simulink model "RocketThrottlingControllersSimulink"  (R2025b)
settings: Solver=ode4  StartTime=0.0  StopTime=6  FixedStep=1e-4  MaxStep=1e-3  RelTol=1e-6
libraries: slpidlib x3, mpclib x2
settings Model: ExtModeTrigDuration=2  Creator=marietakysela  LastModifiedBy=marietakysela
settings SolverCC: AutoInsertRateTranBlk=on
settings OptimizationCC: EnhancedBackFolding=on  PassReuseOutputArgsAs=Individual arguments  ZeroExternalMemoryAtStartup=off  ZeroInternalMemoryAtStartup=off  MaxStackSize=64  OptimizeBlockOrder=speed  DifferentSizesBufferReuse=on  EfficientTunableParamExpr=on
settings DebuggingCC: ParameterTunabilityLossMsg=error
settings HardwareCC: ProdBitPerPointer=32.0  ProdBitPerSizeT=32.0  ProdBitPerPtrDiffT=32.0  ProdLargestAtomicInteger=Long  ProdLargestAtomicFloat=Double  ProdWordSize=32.0  ProdHWDeviceType=ARM Compatible->ARM Cortex  UseEmbeddedCoderFeatures=off  UseSimulinkCoderFeatures=off
settings SFSimCC: MATLABDynamicMemAlloc=off
settings RTWCC: SystemTargetFile=ert.tlc  HardwareBoard=Arduino Uno R4 WiFi  TemplateMakefile=ert_default_tmf  Toolchain=Arduino ARM M4  Description=Embedded Coder
settings CodeAppCC: ForceParamTrailComments=on  IgnoreCustomStorageClasses=off  OperatorAnnotations=on  SimulinkDataObjDesc=on  SFDataObjDesc=on  InsertBlockDesc=on
settings ERTTargetCC: ExtModeTransport=3.0  ExtModeStaticAlloc=on  ExtModeAutomaticAllocSize=off  ExtModeStaticAllocSize=8192.0  ExtModeMexFile=ext_xcp  ExtModeIntrfLevel=Level2 - Open  InlinedParameterPlacement=Hierarchical  SupportContinuousTime=on  SupportNonInlinedSFcns=on  SupportVariableSizeSignals=on

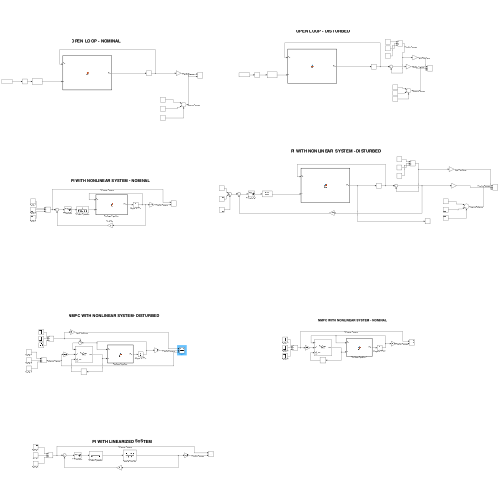
[thumbnail: Simulink's stored preview of the top-level diagram]
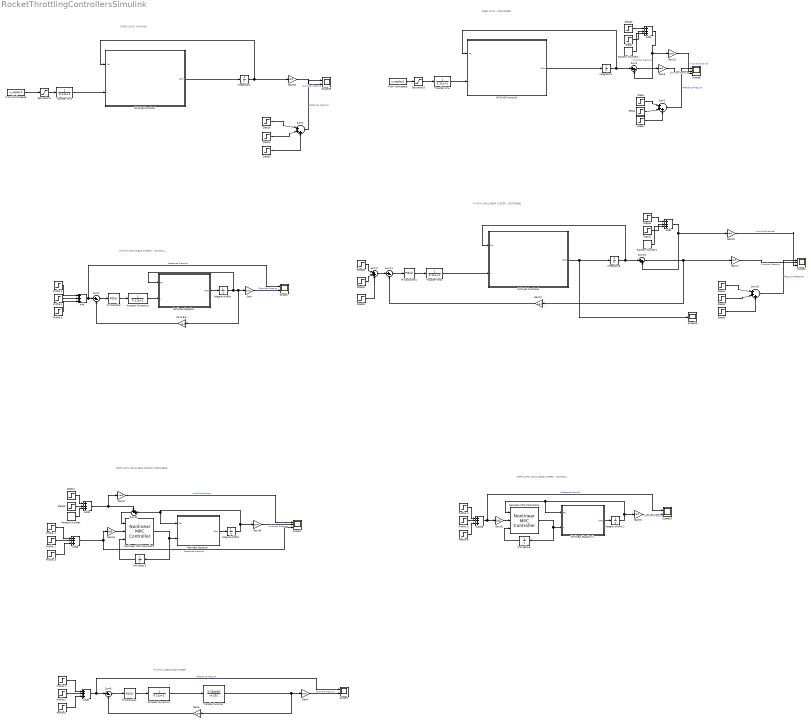
== system RocketThrottlingControllersSimulink ==
  note: PI WITH LINEARIZED SYSTEM
  note: PI WITH NONLINEAR SYSTEM - NOMINAL
  note: OPEN LOOP - DISTURBED
  note: PI WITH NONLINEAR SYSTEM - DISTURBED
  note: NMPC WITH NONLINEAR SYSTEM - NOMINAL
  note: NMPC WITH NONLINEAR SYSTEM- DISTURBED
  note: OPEN LOOP - NOMINAL
  .Integral of dPtc. : Integrator
  Actuator Dynamics : TransferFcn  Denominator=[0.11 1]
  Actuator Dynamics. : TransferFcn  Denominator=[0.11 1]
  Add{,1..2,6,8..9,16} (7 alike) : Sum  Inputs=+++
  From Workspace : FromWorkspace  VariableName=u_replay1
  From Workspace3 : FromWorkspace  VariableName=u_replay1
  Gain{,4..6,11..12,17..18,20..21,30,33} (12 alike) : Gain  Gain=1e-5
  Gain19 : Gain  Gain=1e5
  Gain31 : Gain  Gain=1e5
  Integral of dPtc : Integrator
  Integral of dPtc.2 : Integrator
  Integrator1 : Integrator
  Integrator2 : Integrator
  Integrator6 : Integrator
  MATLAB Function1 : MATLAB Function  TreatAsAtomicUnit=on
  MATLAB Function2 : MATLAB Function  TreatAsAtomicUnit=on
  MATLAB Function6 : MATLAB Function  TreatAsAtomicUnit=on
  "Nonlinear Equation " : MATLAB Function  TreatAsAtomicUnit=on
  Nonlinear Equation. : MATLAB Function  TreatAsAtomicUnit=on
  Nonlinear Equation.1 : MATLAB Function  TreatAsAtomicUnit=on
  Nonlinear MPC Controller3 : mpclib/Nonlinear MPC Controller  nlmpcobj=nlobj  UseObjectTs=on  UseMEX=off  md_enabled=off  mvtarget_enabled=off  param_enabled=off  cost_enabled=off  mvseq_enabled=off  stateseq_enabled=off  ovseq_enabled=off  slack_enabled=off  status_enabled=off  ov_min=off  ov_max=off  mv_min=off  mv_max=off  mvrate_min=off  mvrate_max=off  state_min=off  state_max=off  ov_weight=off  mv_weight=off  mvrate_weight=off  ecr_weight=off  nlp_initialize=off
  Nonlinear MPC Controller6 : mpclib/Nonlinear MPC Controller  nlmpcobj=nlobj  UseObjectTs=on  UseMEX=off  md_enabled=off  mvtarget_enabled=off  param_enabled=off  cost_enabled=off  mvseq_enabled=off  stateseq_enabled=off  ovseq_enabled=off  slack_enabled=off  status_enabled=off  ov_min=off  ov_max=off  mv_min=off  mv_max=off  mvrate_min=off  mvrate_max=off  state_min=off  state_max=off  ov_weight=off  mv_weight=off  mvrate_weight=off  ecr_weight=off  nlp_initialize=off
  PI Controller : slpidlib/PID Controller  Controller=PID  Form=Parallel  TimeDomain=Continuous-time  UseExternalTs=off  SampleTime=-1  IntegratorMethod=Forward Euler  FilterMethod=Forward Euler  ControllerParametersSource=internal  P=0.12  I=0.9  UseKiTs=off  D=0  UseExternalDerivativeSource=off  N=100  UseFilter=on  TunerSelectOption=Frequency Response Based  InitialConditionSource=internal  InitialConditionForIntegrator=0  InitialConditionForFilter=0  DifferentiatorICPrevScaledInput=0  ExternalReset=none  TrackingMode=off  Kt=1  LimitOutput=on  SatLimitsSource=internal  UpperSaturationLimit=0.5  LowerSaturationLimit=0  LinearizeAsGain=on  AntiWindupMode=back-calculation  Kb=8  LimitIntegrator=off  UpperIntegratorSaturationLimit=inf  LowerIntegratorSaturationLimit=-inf  POutMin=[]  POutMax=[]  IOutMin=[]  IOutMax=[]  DOutMin=[]  DOutMax=[]  NOutMin=[]  NOutMax=[]  SumOutMin=[]  SumOutMax=[]  SaturationOutMin=[]  SaturationOutMax=[]  PParamMin=[]  PParamMax=[]  IParamMin=[]  IParamMax=[]  DParamMin=[]  DParamMax=[]  NParamMin=[]  NParamMax=[]  KbParamMin=[]  KbParamMax=[]  KtParamMin=[]  KtParamMax=[]  KbOutMin=[]  KbOutMax=[]  KtOutMin=[]  KtOutMax=[]  IntegratorOutMin=[]  IntegratorOutMax=[]  FilterOutMin=[]  FilterOutMax=[]  SumI1OutMin=[]  SumI1OutMax=[]  SumI2OutMin=[]  SumI2OutMax=[]  SumI3OutMin=[]  SumI3OutMax=[]  SumI4OutMin=[]  SumI4OutMax=[]  SumDOutMin=[]  SumDOutMax=[]  DifferentiatorOutMin=[]  DifferentiatorOutMax=[]  FilterDiffOutCoefMin=[]  FilterDiffOutCoefMax=[]  ReciprocalOutMin=[]  ReciprocalOutMax=[]  SumDenOutMin=[]  SumDenOutMax=[]  SumNumOutMin=[]  SumNumOutMax=[]  DivideOutMin=[]  DivideOutMax=[]  UdiffTsProdOutMin=[]  UdiffTsProdOutMax=[]  NTsProdOutMin=[]  NTsProdOutMax=[]  UintegralTsProdOutMin=[]  UintegralTsProdOutMax=[]  UngainTsProdOutMin=[]  UngainTsProdOutMax=[]  ClampingZeroOutDataTypeStr=Inherit: Inherit via back propagation  ClampingZeroOutMin=[]  ClampingZeroOutMax=[]  FilterDenConstantOutDataTypeStr=Inherit: Inherit via back propagation  FilterDenConstantOutMin=[]  FilterDenConstantOutMax=[]  PCopyOutDataTypeStr=Inherit: Inherit via back propagation  PCopyOutMin=[]  PCopyOutMax=[]  NCopyOutDataTypeStr=Inherit: Inherit via back propagation  NCopyOutMin=[]  NCopyOutMax=[]  IntegratorContinuousStateAttributes=''  IntegratorStateMustResolveToSignalObject=off  IntegratorRTWStateStorageClass=Auto  FilterContinuousStateAttributes=''  FilterStateMustResolveToSignalObject=off  FilterRTWStateStorageClass=Auto  ParallelPVariant=InternalParameters  IdealPVariant=Disabled  IVariant=InternalParameters  DVariant=InternalParameters  IntegratorVariant=Continuous  SatVariant=Enabled  AWVariant=BackCalculation  PCopyVariant=Disabled  TRVariant=Disabled  FdbkBlocksVariant=Forward  IdealPFdbkVariant=Disabled  SatFdbkVariant=Disabled  DerivativeFilterVariant=ContFilter  NVariant=InternalParameters  NCopyVariant=Disabled  FilterICVariant=InternalICsFilter  IntegratorICVariant=InternalICs  ExternalResetVariant=Disabled  TRSumVariant=Passthrough  SumFdbkVariant=Disabled  SumVariant=Sum_PID  TsampFilterVariant=InternalTs  TsampNgainVariant=Passthrough  TsampIntegralVariant=Disabled_SignalSpec  ExternalSaturationOutDataTypeStr=Inherit: Same as second input  DerivativeSourceVariant=ErrorSignal  PreIntVariant=InternalPreInt
  PI Controller. : slpidlib/PID Controller  Controller=PID  Form=Parallel  TimeDomain=Continuous-time  UseExternalTs=off  SampleTime=-1  IntegratorMethod=Forward Euler  FilterMethod=Forward Euler  ControllerParametersSource=internal  P=0.12  I=0.9  UseKiTs=off  D=0  UseExternalDerivativeSource=off  N=100  UseFilter=on  TunerSelectOption=Frequency Response Based  InitialConditionSource=internal  InitialConditionForIntegrator=0  InitialConditionForFilter=0  DifferentiatorICPrevScaledInput=0  ExternalReset=none  TrackingMode=off  Kt=1  LimitOutput=on  SatLimitsSource=internal  UpperSaturationLimit=1  LowerSaturationLimit=0  LinearizeAsGain=on  AntiWindupMode=back-calculation  Kb=9  LimitIntegrator=off  UpperIntegratorSaturationLimit=inf  LowerIntegratorSaturationLimit=-inf  POutMin=[]  POutMax=[]  IOutMin=[]  IOutMax=[]  DOutMin=[]  DOutMax=[]  NOutMin=[]  NOutMax=[]  SumOutMin=[]  SumOutMax=[]  SaturationOutMin=[]  SaturationOutMax=[]  PParamMin=[]  PParamMax=[]  IParamMin=[]  IParamMax=[]  DParamMin=[]  DParamMax=[]  NParamMin=[]  NParamMax=[]  KbParamMin=[]  KbParamMax=[]  KtParamMin=[]  KtParamMax=[]  KbOutMin=[]  KbOutMax=[]  KtOutMin=[]  KtOutMax=[]  IntegratorOutMin=[]  IntegratorOutMax=[]  FilterOutMin=[]  FilterOutMax=[]  SumI1OutMin=[]  SumI1OutMax=[]  SumI2OutMin=[]  SumI2OutMax=[]  SumI3OutMin=[]  SumI3OutMax=[]  SumI4OutMin=[]  SumI4OutMax=[]  SumDOutMin=[]  SumDOutMax=[]  DifferentiatorOutMin=[]  DifferentiatorOutMax=[]  FilterDiffOutCoefMin=[]  FilterDiffOutCoefMax=[]  ReciprocalOutMin=[]  ReciprocalOutMax=[]  SumDenOutMin=[]  SumDenOutMax=[]  SumNumOutMin=[]  SumNumOutMax=[]  DivideOutMin=[]  DivideOutMax=[]  UdiffTsProdOutMin=[]  UdiffTsProdOutMax=[]  NTsProdOutMin=[]  NTsProdOutMax=[]  UintegralTsProdOutMin=[]  UintegralTsProdOutMax=[]  UngainTsProdOutMin=[]  UngainTsProdOutMax=[]  ClampingZeroOutDataTypeStr=Inherit: Inherit via back propagation  ClampingZeroOutMin=[]  ClampingZeroOutMax=[]  FilterDenConstantOutDataTypeStr=Inherit: Inherit via back propagation  FilterDenConstantOutMin=[]  FilterDenConstantOutMax=[]  PCopyOutDataTypeStr=Inherit: Inherit via back propagation  PCopyOutMin=[]  PCopyOutMax=[]  NCopyOutDataTypeStr=Inherit: Inherit via back propagation  NCopyOutMin=[]  NCopyOutMax=[]  IntegratorContinuousStateAttributes=''  IntegratorStateMustResolveToSignalObject=off  IntegratorRTWStateStorageClass=Auto  FilterContinuousStateAttributes=''  FilterStateMustResolveToSignalObject=off  FilterRTWStateStorageClass=Auto  ParallelPVariant=InternalParameters  IdealPVariant=Disabled  IVariant=InternalParameters  DVariant=InternalParameters  IntegratorVariant=Continuous  SatVariant=Enabled  AWVariant=BackCalculation  PCopyVariant=Disabled  TRVariant=Disabled  FdbkBlocksVariant=Forward  IdealPFdbkVariant=Disabled  SatFdbkVariant=Disabled  DerivativeFilterVariant=ContFilter  NVariant=InternalParameters  NCopyVariant=Disabled  FilterICVariant=InternalICsFilter  IntegratorICVariant=InternalICs  ExternalResetVariant=Disabled  TRSumVariant=Passthrough  SumFdbkVariant=Disabled  SumVariant=Sum_PID  TsampFilterVariant=InternalTs  TsampNgainVariant=Passthrough  TsampIntegralVariant=Disabled_SignalSpec  ExternalSaturationOutDataTypeStr=Inherit: Same as second input  DerivativeSourceVariant=ErrorSignal  PreIntVariant=InternalPreInt
  PI Controller1 : slpidlib/PID Controller  Controller=PID  Form=Parallel  TimeDomain=Continuous-time  UseExternalTs=off  SampleTime=-1  IntegratorMethod=Forward Euler  FilterMethod=Forward Euler  ControllerParametersSource=internal  P=0.12  I=0.9  UseKiTs=off  D=0  UseExternalDerivativeSource=off  N=100  UseFilter=on  TunerSelectOption=Transfer Function Based (PID Tuner App)  InitialConditionSource=internal  InitialConditionForIntegrator=0  InitialConditionForFilter=0  DifferentiatorICPrevScaledInput=0  ExternalReset=none  TrackingMode=off  Kt=1  LimitOutput=on  SatLimitsSource=internal  UpperSaturationLimit=0.5  LowerSaturationLimit=0  LinearizeAsGain=on  AntiWindupMode=back-calculation  Kb=8  LimitIntegrator=off  UpperIntegratorSaturationLimit=inf  LowerIntegratorSaturationLimit=-inf  POutMin=[]  POutMax=[]  IOutMin=[]  IOutMax=[]  DOutMin=[]  DOutMax=[]  NOutMin=[]  NOutMax=[]  SumOutMin=[]  SumOutMax=[]  SaturationOutMin=[]  SaturationOutMax=[]  PParamMin=[]  PParamMax=[]  IParamMin=[]  IParamMax=[]  DParamMin=[]  DParamMax=[]  NParamMin=[]  NParamMax=[]  KbParamMin=[]  KbParamMax=[]  KtParamMin=[]  KtParamMax=[]  KbOutMin=[]  KbOutMax=[]  KtOutMin=[]  KtOutMax=[]  IntegratorOutMin=[]  IntegratorOutMax=[]  FilterOutMin=[]  FilterOutMax=[]  SumI1OutMin=[]  SumI1OutMax=[]  SumI2OutMin=[]  SumI2OutMax=[]  SumI3OutMin=[]  SumI3OutMax=[]  SumI4OutMin=[]  SumI4OutMax=[]  SumDOutMin=[]  SumDOutMax=[]  DifferentiatorOutMin=[]  DifferentiatorOutMax=[]  FilterDiffOutCoefMin=[]  FilterDiffOutCoefMax=[]  ReciprocalOutMin=[]  ReciprocalOutMax=[]  SumDenOutMin=[]  SumDenOutMax=[]  SumNumOutMin=[]  SumNumOutMax=[]  DivideOutMin=[]  DivideOutMax=[]  UdiffTsProdOutMin=[]  UdiffTsProdOutMax=[]  NTsProdOutMin=[]  NTsProdOutMax=[]  UintegralTsProdOutMin=[]  UintegralTsProdOutMax=[]  UngainTsProdOutMin=[]  UngainTsProdOutMax=[]  ClampingZeroOutDataTypeStr=Inherit: Inherit via back propagation  ClampingZeroOutMin=[]  ClampingZeroOutMax=[]  FilterDenConstantOutDataTypeStr=Inherit: Inherit via back propagation  FilterDenConstantOutMin=[]  FilterDenConstantOutMax=[]  PCopyOutDataTypeStr=Inherit: Inherit via back propagation  PCopyOutMin=[]  PCopyOutMax=[]  NCopyOutDataTypeStr=Inherit: Inherit via back propagation  NCopyOutMin=[]  NCopyOutMax=[]  IntegratorContinuousStateAttributes=''  IntegratorStateMustResolveToSignalObject=off  IntegratorRTWStateStorageClass=Auto  FilterContinuousStateAttributes=''  FilterStateMustResolveToSignalObject=off  FilterRTWStateStorageClass=Auto  ParallelPVariant=InternalParameters  IdealPVariant=Disabled  IVariant=InternalParameters  DVariant=InternalParameters  IntegratorVariant=Continuous  SatVariant=Enabled  AWVariant=BackCalculation  PCopyVariant=Disabled  TRVariant=Disabled  FdbkBlocksVariant=Forward  IdealPFdbkVariant=Disabled  SatFdbkVariant=Disabled  DerivativeFilterVariant=ContFilter  NVariant=InternalParameters  NCopyVariant=Disabled  FilterICVariant=InternalICsFilter  IntegratorICVariant=InternalICs  ExternalResetVariant=Disabled  TRSumVariant=Passthrough  SumFdbkVariant=Disabled  SumVariant=Sum_PID  TsampFilterVariant=InternalTs  TsampNgainVariant=Passthrough  TsampIntegralVariant=Disabled_SignalSpec  ExternalSaturationOutDataTypeStr=Inherit: Same as second input  DerivativeSourceVariant=ErrorSignal  PreIntVariant=InternalPreInt
  Pa to Bar : Gain  Gain=1e-5
  Profile 1 : Step  Before=1.01  After=10  SampleTime=0
  Profile 1. : Step  After=10  SampleTime=0
  Profile 2 : Step  Time=4  After=15  SampleTime=0
  Profile 2. : Step  Time=4  After=15  SampleTime=0
  Profile 3 : Step  Time=3  After=-5  SampleTime=0
  Profile 3. : Step  Time=3  After=-5  SampleTime=0
  Profile. 1 : Step  Before=1.01  After=10  SampleTime=0
  Profile. 2 : Step  Time=4  After=15  SampleTime=0
  Profile. 3 : Step  Time=3  After=-5  SampleTime=0
  Profile. 4 : Step  Before=1.01  After=10  SampleTime=0
  Profile. 5 : Step  Time=4  After=15  SampleTime=0
  Profile. 6 : Step  Time=3  After=-5  SampleTime=0
  Random Number : RandomNumber  Variance=5e8  SampleTime=0.01
  Random Number1 : RandomNumber  Variance=5e8  SampleTime=0.01
  Random Number2 : RandomNumber  Variance=5e8  SampleTime=0.01
  Saturation1 : Saturate  UpperLimit=0.8  LowerLimit=0
  Saturation3 : Saturate  UpperLimit=0.8  LowerLimit=0
  Scope{2,6,19,28} (4 alike) : Scope  NumInputPorts=2
      Scope19 settings: TimeUnits=Metric (based on Time Span)  Title=Reference vs Chamber Pressure with NMPC  ActiveDisplayYMinimum=-2.4999999999999996  ActiveDisplayYMaximum=22.5  YLabel=Pressure (Bar)  DataLoggingVariableName=ScopeData19
      Scope2 settings: TimeUnits=Metric (based on Time Span)  Title=Reference vs Chamber Pressure  ActiveDisplayYMinimum=-2.4999999999999996  ActiveDisplayYMaximum=22.5  YLabel=Pressure (Bar)  DataLoggingVariableName=ScopeData2
      Scope28 settings: TimeUnits=Metric (based on Time Span)  Title=Reference vs Chamber Pressure  ActiveDisplayYMinimum=-2.4999999999999996  ActiveDisplayYMaximum=22.5  YLabel=Pressure (Bar)  DataLoggingVariableName=ScopeData28
      Scope6 settings: TimeUnits=Metric (based on Time Span)  Title=Linearized System Reference vs Chamber Pressure  ActiveDisplayYMinimum=-2.4999999999999996  ActiveDisplayYMaximum=22.5  YLabel=Pressure (Bar)  DataLoggingVariableName=ScopeData6
  Scope23 : Scope
      settings: ActiveDisplayYMinimum=-116.22763400424904  ActiveDisplayYMaximum=176.07208701829447  DataLoggingVariableName=ScopeData23
  Scope4 : Scope  NumInputPorts=3
      settings: TimeUnits=Metric (based on Time Span)  Title=Reference vs Disturbed Chamber Pressure with PI  ActiveDisplayYMinimum=-3.3034504728865297  ActiveDisplayYMaximum=23.307387134551131  YLabel=Pressure (Bar)
  Scope7 : Scope  NumInputPorts=3
      settings: TimeUnits=Metric (based on Time Span)  Title=Reference vs Disturbed Chamber Pressure with NMPC  ActiveDisplayYMinimum=7.5474967168474105  ActiveDisplayYMaximum=11.712992718191334  YLabel=Pressure (Bar)  DataLoggingVariableName=ScopeData7
  Scope8 : Scope  NumInputPorts=3
      settings: TimeUnits=Metric (based on Time Span)  Title=Reference vs Disturbed Chamber Pressure without Control  ActiveDisplayYMinimum=-3.3049105304961062  ActiveDisplayYMaximum=23.32052765303732  YLabel=Pressure (Bar)  DataLoggingVariableName=ScopeData3
  Step12 : Step  Time=2  After=-2e5  SampleTime=0
  Step13 : Step  Time=2.5  After=2e5  SampleTime=0
  Step19 : Step  Before=1.01  After=10  SampleTime=0
  Step22 : Step  Time=2.5  After=2e5  SampleTime=0
  Step23 : Step  Time=2  After=-2e5  SampleTime=0
  Step{4,24,40,42} (4 alike) : Step  Time=4  After=15  SampleTime=0
  Step3 : Step  After=10  SampleTime=0
  Step{5,33,39,43} (4 alike) : Step  Time=3  After=-5  SampleTime=0
  Step38 : Step  Before=1.01  After=10  SampleTime=0
  Step41 : Step  After=10  SampleTime=0
  Step44 : Step  Time=2  After=-2e5  SampleTime=0
  Step6 : Step  Time=2.5  After=2e5  SampleTime=0
  Sum1 : Sum  Inputs=|+-
  Sum14 : Sum  Inputs=|+-
  Sum{2,5,17..18} (4 alike) : Sum  Inputs=|+++
  Sum19 : Sum  Inputs=|++
  Sum23 : Sum  Inputs=++|
  Sum3 : Sum  Inputs=|++
  Sum6 : Sum  Inputs=|+-
  Transfer Fcn1 : TransferFcn  Denominator=[0.11 1]
  Transfer Fcn4 : TransferFcn  Denominator=[0.11 1]
  Transfer Fcn8 : TransferFcn  Denominator=[0.11 1]
  Transfer Function : TransferFcn  Numerator=[9.338e08]  Denominator=[1 252]
  Unit Delay3 : UnitDelay  InitialCondition=0.3  SampleTime=-1  HasFrameUpgradeWarning=on
  Unit Delay6 : UnitDelay  InitialCondition=0.3  SampleTime=-1  HasFrameUpgradeWarning=on
  wires:
  Profile 1/1 -> Add/1
  Profile 2/1 -> Add/2
  Add/1 -> Sum1/1, Scope2/1  "Reference Pressure"
  Pa to Bar/1 -> Sum1/2
  Profile 3/1 -> Add/3
  Add6/1 -> Scope6/1, Sum6/1  "Reference Pressure"
  Gain5/1 -> Sum6/2
  Actuator Dynamics./1 -> Transfer Function/1
  Saturation3/1 -> Transfer Fcn4/1
  MATLAB Function2/1(dPtc) -> Integrator2/1
  "Nonlinear Equation "/1(dPtc) -> Integral of dPtc/1
  Gain6/1 -> Scope8/2  "Chamber Pressure"
  Gain11/1 -> Scope4/2  "Chamber Pressure"
  Sum18/1 -> Scope4/1  "Pressure Reference"
  Integrator6/1 -> MATLAB Function6/1(Ptc), Sum19/1
  Step38/1 -> Sum17/1
  Step41/1 -> Sum18/1
  Sum14/1 -> PI Controller1/1
  Step40/1 -> Sum17/2
  Step42/1 -> Sum18/2
  Gain12/1 -> Sum14/2
  Step43/1 -> Sum18/3
  MATLAB Function6/1(dPtc) -> Integrator6/1, Scope23/1
  Step39/1 -> Sum17/3
  Sum17/1 -> Sum14/1
  Transfer Function/1 -> Gain5/1, Gain4/1
  Sum19/1 -> Gain12/1, Gain11/1
  Gain/1 -> Scope2/2  "Chamber Pressure"
  PI Controller1/1 -> Transfer Fcn8/1
  Integral of dPtc/1 -> Pa to Bar/1, Gain/1, "Nonlinear Equation "/1(Ptc)
  PI Controller/1 -> Actuator Dynamics/1
  Sum1/1 -> PI Controller/1
  PI Controller./1 -> Actuator Dynamics./1
  Sum6/1 -> PI Controller./1
  Step5/1 -> Sum2/3
  Step4/1 -> Sum2/2
  Sum2/1 -> Scope8/1  "Reference Pressure"
  Step3/1 -> Sum2/1
  Integrator2/1 -> Sum3/1, MATLAB Function2/1(Ptc)
  From Workspace/1 -> Saturation3/1
  Transfer Fcn4/1 -> MATLAB Function2/2(u)
  Step44/1 -> Add1/1
  Step22/1 -> Add1/2
  Add1/1 -> Sum19/2, Gain20/1
  Step6/1 -> Add2/2
  Step23/1 -> Add2/1
  Sum3/1 -> Gain6/1
  Profile 1./1 -> Add6/1
  Profile 3./1 -> Add6/3
  Profile 2./1 -> Add6/2
  Gain4/1 -> Scope6/2  "Chamber Pressure"
  Step13/1 -> Add9/2
  Sum23/1 -> Nonlinear MPC Controller3/1
  Add9/1 -> Gain17/1, Sum23/1
  Nonlinear Equation./1(dPtc) -> .Integral of dPtc./1
  Gain18/1 -> Scope7/2  "Chamber Pressure"
  Profile. 2/1 -> Add8/2
  Unit Delay3/1 -> Nonlinear MPC Controller3/3
  Gain19/1 -> Nonlinear MPC Controller3/2
  Gain17/1 -> Scope7/1  "Input Disturbance"
  Profile. 3/1 -> Add8/3
  Step12/1 -> Add9/1
  Profile. 1/1 -> Add8/1
  Add8/1 -> Scope7/3, Gain19/1  "Reference Pressure"
  .Integral of dPtc./1 -> Gain18/1, Nonlinear Equation./1(Ptc), Sum23/2
  Nonlinear MPC Controller3/1 -> Unit Delay3/1, Nonlinear Equation./2(u)
  Random Number1/1 -> Add1/3
  Gain20/1 -> Scope4/3  "Input Disturbance"
  Random Number2/1 -> Add2/3
  Add2/1 -> Sum3/2, Gain21/1  "Chamber Pressure"
  Gain21/1 -> Scope8/3  "Input Disturbance"
  Random Number/1 -> Add9/3
  Transfer Fcn8/1 -> MATLAB Function6/2(u)
  Actuator Dynamics/1 -> "Nonlinear Equation "/2(u)
  Gain30/1 -> Scope19/2  "Chamber Pressure"
  Profile. 6/1 -> Add16/3
  Profile. 5/1 -> Add16/2
  Add16/1 -> Scope19/1, Gain31/1  "Reference Pressure"
  Profile. 4/1 -> Add16/1
  Nonlinear MPC Controller6/1 -> Unit Delay6/1, Nonlinear Equation.1/2(u)
  Gain31/1 -> Nonlinear MPC Controller6/2
  Integral of dPtc.2/1 -> Gain30/1, Nonlinear Equation.1/1(Ptc), Nonlinear MPC Controller6/1
  Nonlinear Equation.1/1(dPtc) -> Integral of dPtc.2/1
  Unit Delay6/1 -> Nonlinear MPC Controller6/3
  Transfer Fcn1/1 -> MATLAB Function1/2(u)
  Step19/1 -> Sum5/1
  MATLAB Function1/1(dPtc) -> Integrator1/1
  From Workspace3/1 -> Saturation1/1
  Integrator1/1 -> Gain33/1, MATLAB Function1/1(Ptc)
  Sum5/1 -> Scope28/1  "Reference Pressure"
  Saturation1/1 -> Transfer Fcn1/1
  Gain33/1 -> Scope28/2  "Chamber Pressure"
  Step33/1 -> Sum5/3
  Step24/1 -> Sum5/2

== matlab function RocketThrottlingControllersSimulink/Nonlinear Equation  ==
  data: Ptc input; u input; dPtc output
function dPtc = fcn(Ptc,u)
% where u = mdot_o


R = 282;
Tc = 3000; 
ao = 2.93e-4;
n = 0.518;
Vc = 9.5e-4;
r = 0.01;
Lf = 0.315;
rhof = 900;
gamma = 1.13;
nc = 0.7;
Cd = 1;
Ath = (pi*0.02^2)/4;

K1 = (R*Tc)/Vc;
K2 = 2*pi*r*Lf*ao;
K3 = rhof;
K4 = R*Tc;
choked = (2/(gamma+1))^((gamma+1)/(2*(gamma-1)));
K5 = (gamma*Cd*Ath)/(nc*sqrt(gamma*R*Tc)) * choked;
u_eff = max(u,0);        
u_n   = u_eff.^n;
dPtc = K1*((K2/(pi*r^2)^n)*(u_n)*(K3-(Ptc/K4)) + u_eff - K5*Ptc);

== matlab function RocketThrottlingControllersSimulink/MATLAB Function2 ==
  data: Ptc input; u input; dPtc output
function dPtc = fcn(Ptc,u)
% where u = mdot_o


R = 282;
Tc = 3000; 
ao = 2.93e-4;
n = 0.518;
Vc = 9.5e-4;
r = 0.01;
Lf = 0.315;
rhof = 900;
gamma = 1.13;
nc = 0.7;
Cd = 1;
Ath = (pi*0.02^2)/4;

K1 = (R*Tc)/Vc;
K2 = 2*pi*r*Lf*ao;
K3 = rhof;
K4 = R*Tc;
choked = (2/(gamma+1))^((gamma+1)/(2*(gamma-1)));
K5 = (gamma*Cd*Ath)/(nc*sqrt(gamma*R*Tc)) * choked;
dPtc = K1*((K2/(pi*r^2)^n)*(u.^n)*(K3-(Ptc/K4))+u-K5*Ptc);

== matlab function RocketThrottlingControllersSimulink/MATLAB Function6 ==
  data: Ptc input; u input; dPtc output
function dPtc = fcn(Ptc,u)
% where u = mdot_o


R = 282;
Tc = 2500; 
ao = 2.93e-4;
n = 0.518;
Vc = 9.5e-4;
r = 0.01;
Lf = 0.315;
rhof = 900;
gamma = 1.13;
nc = 0.7;
Cd = 1;
Ath = (pi*0.02^2)/4;

K1 = (R*Tc)/Vc;
K2 = 2*pi*r*Lf*ao;
K3 = rhof;
K4 = R*Tc;
choked = (2/(gamma+1))^((gamma+1)/(2*(gamma-1)));
K5 = (gamma*Cd*Ath)/(nc*sqrt(gamma*R*Tc)) * choked;
dPtc = K1*((K2/(pi*r^2)^n)*(u.^n)*(K3-(Ptc/K4))+u-K5*Ptc);

== matlab function RocketThrottlingControllersSimulink/Nonlinear Equation. ==
  data: Ptc input; u input; dPtc output
function dPtc = fcn(Ptc,u)
% where u = mdot_o


R = 282;
Tc = 3000; 
ao = 2.93e-4;
n = 0.518;
Vc = 9.5e-4;
r = 0.01;
Lf = 0.315;
rhof = 900;
gamma = 1.13;
nc = 0.7;
Cd = 1;
Ath = (pi*0.02^2)/4;

K1 = (R*Tc)/Vc;
K2 = (2*pi*r*Lf*ao);
K3 = rhof;
K4 = R*Tc;
choked = (2/(gamma+1))^((gamma+1)/(2*(gamma-1)));
K5 = (gamma*Cd*Ath)/(nc*sqrt(gamma*R*Tc)) * choked;
dPtc = K1*((K2/(pi*r^2)^n)*(u.^n)*(K3-(Ptc/K4))+u-K5*Ptc);

== matlab function RocketThrottlingControllersSimulink/Nonlinear Equation.1 ==
  data: Ptc input; u input; dPtc output
function dPtc = fcn(Ptc,u)
% where u = mdot_o


R = 282;
Tc = 3000; 
ao = 2.93e-4;
n = 0.518;
Vc = 9.5e-4;
r = 0.01;
Lf = 0.315;
rhof = 900;
gamma = 1.13;
nc = 0.7;
Cd = 1;
Ath = (pi*0.02^2)/4;

K1 = (R*Tc)/Vc;
K2 = (2*pi*r*Lf*ao);
K3 = rhof;
K4 = R*Tc;
choked = (2/(gamma+1))^((gamma+1)/(2*(gamma-1)));
K5 = (gamma*Cd*Ath)/(nc*sqrt(gamma*R*Tc)) * choked;
dPtc = K1*((K2/(pi*r^2)^n)*(u.^n)*(K3-(Ptc/K4))+u-K5*Ptc);

== matlab function RocketThrottlingControllersSimulink/MATLAB Function1 ==
  data: Ptc input; u input; dPtc output
function dPtc = fcn(Ptc,u)
% where u = mdot_o


R = 282;
Tc = 3000; 
ao = 2.93e-4;
n = 0.518;
Vc = 9.5e-4;
r = 0.01;
Lf = 0.315;
rhof = 900;
gamma = 1.13;
nc = 0.7;
Cd = 1;
Ath = (pi*0.02^2)/4;

K1 = (R*Tc)/Vc;
K2 = 2*pi*r*Lf*ao;
K3 = rhof;
K4 = R*Tc;
choked = (2/(gamma+1))^((gamma+1)/(2*(gamma-1)));
K5 = (gamma*Cd*Ath)/(nc*sqrt(gamma*R*Tc)) * choked;
dPtc = K1*((K2/(pi*r^2)^n)*(u.^n)*(K3-(Ptc/K4))+u-K5*Ptc);
